simulink model "modelPoruchaCtyrka"  (R2016a)
settings: Solver=FixedStepAuto  StartTime=0.0  StopTime=100  FixedStep=0.0001  MaxStep=1e-2  RelTol=1e-3
settings Model: Creator=NTB  LastModifiedBy=Jan
settings DataIOCC: LimitDataPoints=on  SaveFormat=Array
settings OptimizationCC: ExpressionDepthLimit=2147483647
settings DebuggingCC: UnderspecifiedInitializationDetection=Classic  MergeDetectMultiDrivingBlocksExec=none  SolverPrmCheckMsg=warning  StateNameClashWarn=warning
settings HardwareCC: ProdBitPerPointer=32  ProdLargestAtomicFloat=None  ProdIntDivRoundTo=Undefined  ProdEndianess=Unspecified  ProdWordSize=32  ProdHWDeviceType=32-bit Generic
settings ModelReferenceCC: PropagateSignalLabelsOutOfModel=off
settings ConfigComp: CovModelRefEnable=Off

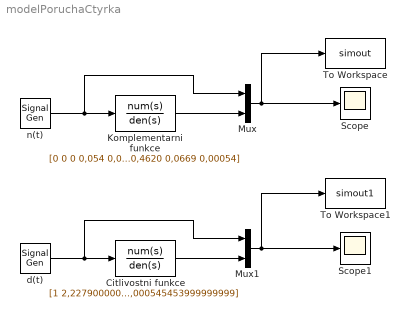
== system modelPoruchaCtyrka ==
  Citlivostni funkce : TransferFcn  Numerator=[1 2,22790000000000 0,462000000000000 0,0124000000000000 0]  Denominator=[1 2,22790000000000 0,462000000000000 0,0669453999999999 0,000545453999999999]
  Komplementarni funkce : TransferFcn  Numerator=[0 0 0 0,054 0,00054]  Denominator=[1 2,2270,4620 0,0669 0,00054]
  Mux : Mux  Inputs=2
  Mux1 : Mux  Inputs=2
  Scope : Scope
  Scope1 : Scope
  To Workspace : ToWorkspace  VariableName=simout  SaveFormat=Timeseries  SampleTime=-1
  To Workspace1 : ToWorkspace  VariableName=simout1  SaveFormat=Timeseries  SampleTime=-1
  d(t) : SignalGenerator  Frequency=0.21  Units=rad/sec
  n(t) : SignalGenerator  Frequency=0.12  Units=rad/sec
  wires:
  Mux/1 -> To Workspace/1, Scope/1
  Komplementarni funkce/1 -> Mux/2
  n(t)/1 -> Mux/1, Komplementarni funkce/1
  Mux1/1 -> To Workspace1/1, Scope1/1
  Citlivostni funkce/1 -> Mux1/2
  d(t)/1 -> Mux1/1, Citlivostni funkce/1
